simulink model "Double_mass_integrator_method"  (R2024a)
settings: Solver=VariableStepAuto  StartTime=0.0  StopTime=10.0  RelTol=1e-3
values from neighbouring files (symbols this model uses):
  b1 = 1    [Double_mass_parameters.mat]
  b2 = 1    [Double_mass_parameters.mat]
  k1 = 100    [Double_mass_parameters.mat]
  k2 = 10000    [Double_mass_parameters.mat]
  m1 = 25    [Double_mass_parameters.mat]
  m2 = 1    [Double_mass_parameters.mat]
settings Model: Creator=nassa  LastModifiedBy=nassa

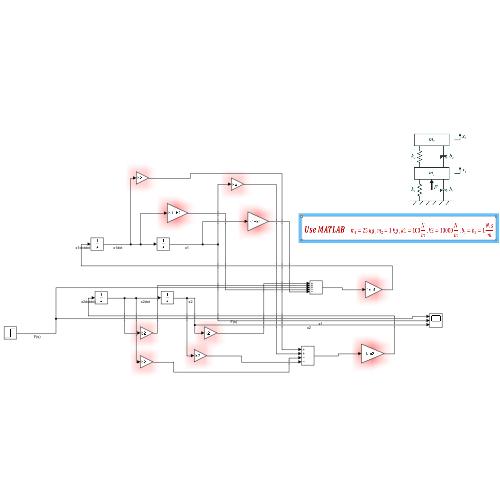
[thumbnail: Simulink's stored preview of the top-level diagram]
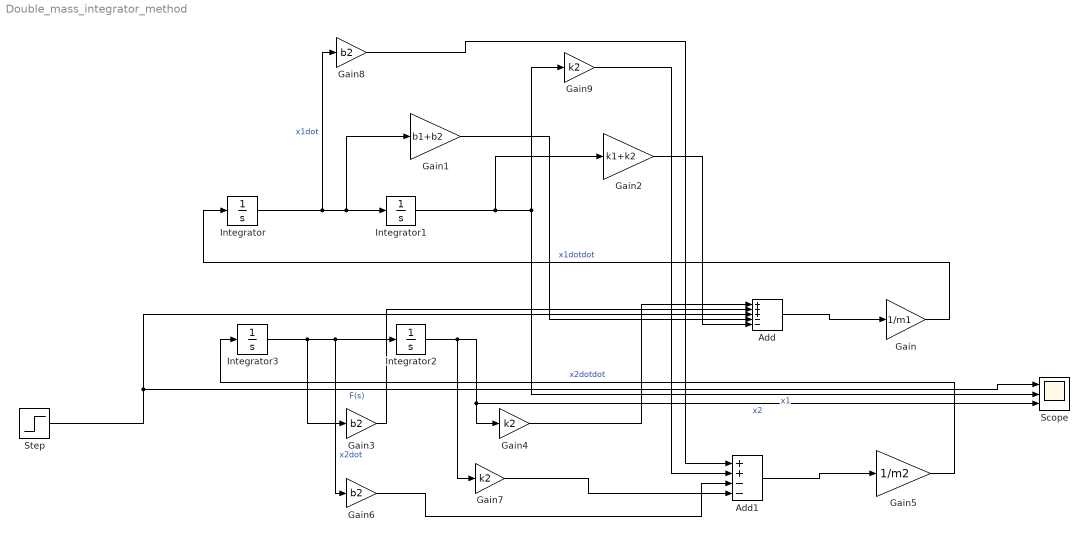
== system Double_mass_integrator_method ==
  Add : Sum  Inputs=+++--
  Add1 : Sum  Inputs=++--
  Gain : Gain  Gain=1/m1
  Gain1 : Gain  Gain=b1+b2
  Gain2 : Gain  Gain=k1+k2
  Gain3 : Gain  Gain=b2
  Gain4 : Gain  Gain=k2
  Gain5 : Gain  Gain=1/m2
  Gain6 : Gain  Gain=b2
  Gain7 : Gain  Gain=k2
  Gain8 : Gain  Gain=b2
  Gain9 : Gain  Gain=k2
  Integrator{,1..3} (4 alike) : Integrator
  Scope : Scope  NumInputPorts=3
  Step : Step  SampleTime=0
  wires:
  Integrator3/1 -> Gain3/1, Gain6/1, Integrator2/1  "x2dot"
  Integrator/1 -> Gain8/1, Gain1/1, Integrator1/1  "x1dot"
  Gain/1 -> Integrator/1  "x1dotdot"
  Integrator1/1 -> Scope/2, Gain9/1, Gain2/1  "x1"
  Gain5/1 -> Integrator3/1  "x2dotdot"
  Integrator2/1 -> Gain7/1, Scope/3, Gain4/1  "x2"
  Gain4/1 -> Add/1
  Gain3/1 -> Add/2
  Step/1 -> Scope/1, Add/3  "F(s)"
  Gain1/1 -> Add/4
  Gain2/1 -> Add/5
  Add/1 -> Gain/1
  Gain8/1 -> Add1/1
  Gain9/1 -> Add1/2
  Gain6/1 -> Add1/3
  Gain7/1 -> Add1/4
  Add1/1 -> Gain5/1
